simulink model "Mission_Manager_HIL"  (R2025b)
settings: Solver=FixedStepDiscrete  StartTime=0.0  StopTime=tspan  FixedStep=dt_sim  RelTol=1e-3
undefined symbols (not defined in the file): dt_control, dt_data, pwm_zero_set
libraries: ros2lib x7
settings Model: Creator=vulcangrip  LastModifiedBy=kjhaydon
settings OptimizationCC: DefaultParameterBehavior=Inlined  EnhancedBackFolding=on  PassReuseOutputArgsAs=Individual arguments  ZeroExternalMemoryAtStartup=off  ZeroInternalMemoryAtStartup=off  MaxStackSize=64  OptimizeBlockOrder=speed  DifferentSizesBufferReuse=on  OptimizationCustomize=off  EfficientTunableParamExpr=on
settings DebuggingCC: ParameterTunabilityLossMsg=error
settings HardwareCC: ProdBitPerLong=64.0  ProdHWDeviceType=Intel->x86-64 (Linux 64)
settings SFSimCC: MATLABDynamicMemAlloc=off  SimTargetLang=C++  SimDLTargetLibrary=mkl-dnn
settings RTWCC: SystemTargetFile=ert.tlc  HardwareBoard=Robot Operating System 2 (ROS 2)  TLCOptions="-aInlineSetEventsForThisBaseRateFcn=TLC_FALSE -aSuppressMultiTaskScheduler=TLC_FALSE  -aRateBasedStepFcn=0"  GenCodeOnly=on  TemplateMakefile=ert_default_tmf  Toolchain=Colcon Tools  TargetLang=C++  CheckMdlBeforeBuild=Warning  Description=Embedded Coder
settings CodeAppCC: ForceParamTrailComments=on  IgnoreCustomStorageClasses=off  OperatorAnnotations=on  SimulinkDataObjDesc=on  SFDataObjDesc=on  InsertBlockDesc=on
settings ERTTargetCC: ExtModeTransport=2.0  ExtModeStaticAlloc=on  ExtModeAutomaticAllocSize=off  ExtModeMexFile=ext_xcp  ExtModeIntrfLevel=Level2 - Open  RootIOFormat=Structure reference  TargetLangStandard=C++11 (ISO)  CodeInterfacePackaging=C++ class  SubcomponentCodeInterfacePackaging=C++ class

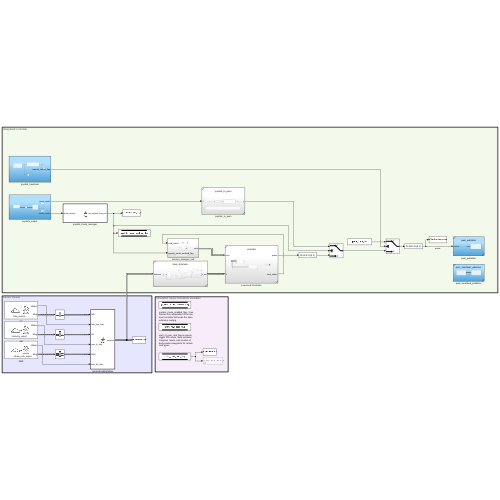
[thumbnail: Simulink's stored preview of the top-level diagram]
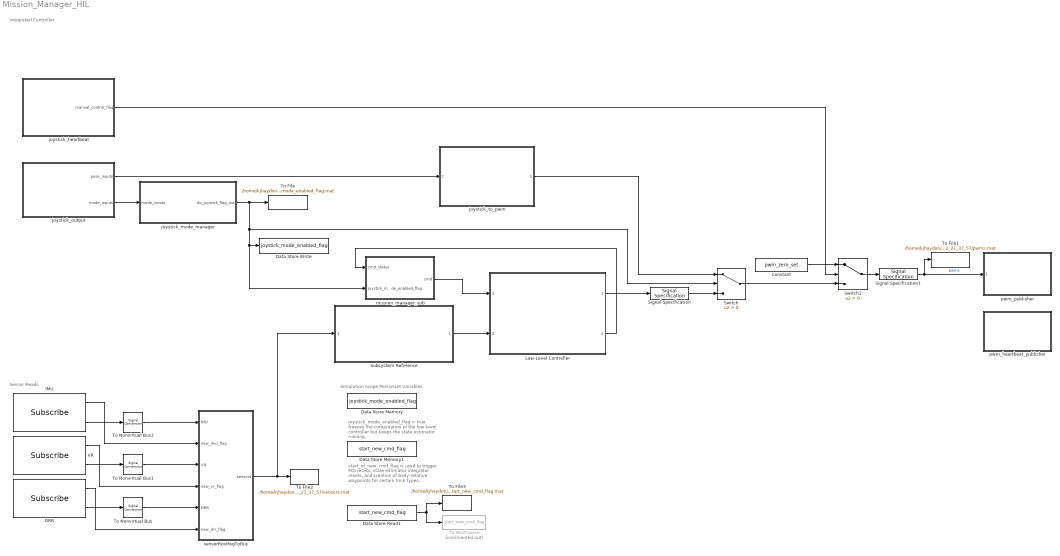
== system Mission_Manager_HIL ==
  note: Integrated Controller
  note: Sensor Reads
  note: Simulation Scope Persistant Variables
  note: joystick_mode_enabled_flag = true freezes the computation of the low-level controller but keeps the state estimator running.
  note: start_of_new_cmd_flag is used to trigger PID resets, state estimator integrator resets, and creation of body-relative waypoints for certain trick types.
  Constant : Constant  Value=pwm_zero_set  OutDataTypeStr=int32
  DRR : ros2lib/Subscribe  topicSource=Select from ROS network  topic=/dead_reck_report  messageType=custom_interfaces/DRR  sampleTime=-1  QOSHistory=Keep last  QOSDepth=10  QOSReliability=Reliable  QOSDurability=Volatile  QOSDeadline=Inf  QOSLifespan=Inf  QOSLiveliness=Automatic  QOSLeaseDuration=Inf  QOSAvoidROSNamespaceConventions=off
  Data Store Memory : DataStoreMemory  DataStoreName=joystick_mode_enabled_flag  WriteAfterWriteMsg=warning  InitialValue=initial_joystick_mode_enabled_flag  ShowAdditionalParam=off  OutDataTypeStr=boolean
  Data Store Memory1 : DataStoreMemory  DataStoreName=start_new_cmd_flag  WriteAfterWriteMsg=warning  InitialValue=true  ShowAdditionalParam=off  OutDataTypeStr=boolean
  Data Store Read1 : DataStoreRead  DataStoreName=start_new_cmd_flag  IndexOptions=Index vector (dialog)  Indices=1  OutputSizes=1
  Data Store Write : DataStoreWrite  DataStoreName=joystick_mode_enabled_flag  SampleTime=dt_control  IndexOptions=Index vector (dialog)  Indices=1  OutputSizes=1
  IMU : ros2lib/Subscribe  topicSource=Specify your own  topic=/imu_custom  messageType=custom_interfaces/Imu  sampleTime=1/100  QOSHistory=Keep last  QOSDepth=10  QOSReliability=Reliable  QOSDurability=Volatile  QOSDeadline=Inf  QOSLifespan=Inf  QOSLiveliness=Automatic  QOSLeaseDuration=Inf  QOSAvoidROSNamespaceConventions=off
  Low-Level Controller : Subsystem  ReferencedSubsystem=controller
  Signal Specification : SignalSpecification  OutDataTypeStr=int32  Dimensions=[8 1]
  Signal Specification1 : SignalSpecification  OutDataTypeStr=int32  Dimensions=[8 1]
  Subsystem Reference : Subsystem  ReferencedSubsystem=State_Estimator
  Switch : Switch  Criteria=u2 > Threshold  SaturateOnIntegerOverflow=off  InputSameDT=off
  Switch1 : Switch  Criteria=u2 > Threshold  SaturateOnIntegerOverflow=off  InputSameDT=off
  To File : ToFile  Filename=/home/kjhaydon/Github/Robosub/SimulinkPlant/data/2026_06_22_21_37_57/joystick_mode_enabled_flag.mat  MatrixName=joystick_mode_enabled_flag  SaveFormat=Timeseries  SampleTime=dt_control
  To File1 : ToFile  Filename=/home/kjhaydon/Github/Robosub/SimulinkPlant/data/2026_06_22_21_37_57/pwms.mat  MatrixName=pwms  SaveFormat=Timeseries  SampleTime=dt_control
  To File2 : ToFile  Filename=/home/kjhaydon/Github/Robosub/SimulinkPlant/data/2026_06_22_21_37_57/sensors.mat  MatrixName=sensors  SaveFormat=Timeseries
  To File3 : ToFile  Filename=/home/kjhaydon/Github/Robosub/SimulinkPlant/data/2026_06_22_21_37_57/start_new_cmd_flag.mat  MatrixName=start_new_cmd_flag  SaveFormat=Timeseries
  To Nonvirtual Bus : SignalConversion  ConversionOutput=Nonvirtual bus  OutDataTypeStr=Bus: SL_Bus_custom_interfaces_DRR  OverrideOpt=off
  To Nonvirtual Bus1 : SignalConversion  ConversionOutput=Nonvirtual bus  OutDataTypeStr=Bus: SL_Bus_custom_interfaces_VR  OverrideOpt=off
  To Nonvirtual Bus2 : SignalConversion  ConversionOutput=Nonvirtual bus  OutDataTypeStr=Bus: SL_Bus_custom_interfaces_Imu  OverrideOpt=off
  To Workspace : ToWorkspace  Commented=on  VariableName=start_new_cmd_flag  SaveFormat=Timeseries  SampleTime=dt_data
  VR : ros2lib/Subscribe  topicSource=Select from ROS network  topic=/velocity_report  messageType=custom_interfaces/VR  sampleTime=-1  QOSHistory=Keep last  QOSDepth=10  QOSReliability=Reliable  QOSDurability=Volatile  QOSDeadline=Inf  QOSLifespan=Inf  QOSLiveliness=Automatic  QOSLeaseDuration=Inf  QOSAvoidROSNamespaceConventions=off
  joystick_heartbeat : Subsystem
  joystick_mode_manager : MATLAB Function  TreatAsAtomicUnit=on
  joystick_output : Subsystem
  joystick_to_pwm : Subsystem  ReferencedSubsystem=joystick_to_pwm
  mission_manager_sub : Subsystem
  pwm_heartbeat_publisher : Subsystem  ReferencedSubsystem=pwm_heartbeat_publisher
  pwm_publisher : Subsystem  ReferencedSubsystem=pwm_publisher
  sensorRosMsgToBus : MATLAB Function  TreatAsAtomicUnit=on
  wires:
  IMU/2 -> To Nonvirtual Bus2/1
  DRR/2 -> To Nonvirtual Bus/1
  VR/2 -> To Nonvirtual Bus1/1
  joystick_output/2(mode_inputs) -> joystick_mode_manager/1(mode_inputs)
  mission_manager_sub/1(cmd) -> Low-Level Controller/1
  Low-Level Controller/2 -> mission_manager_sub/1(cmd_status)
  Low-Level Controller/1 -> Signal Specification/1
  joystick_to_pwm/1 -> Switch/1
  Signal Specification/1 -> Switch/3
  joystick_output/1(pose_inputs) -> joystick_to_pwm/1
  Subsystem Reference/1 -> Low-Level Controller/2
  To Nonvirtual Bus1/1 -> sensorRosMsgToBus/3(VR)
  To Nonvirtual Bus/1 -> sensorRosMsgToBus/5(DRR)
  sensorRosMsgToBus/1(sensors) -> Subsystem Reference/1, To File2/1
  joystick_mode_manager/1(do_joystick_flag_out) -> mission_manager_sub/2(joystick_mode_enabled_flag), Data Store Write/1, Switch/2, To File/1
  Signal Specification1/1 -> To File1/1, pwm_publisher/1  "pwms"
  To Nonvirtual Bus2/1 -> sensorRosMsgToBus/1(IMU)
  Data Store Read1/1 -> To File3/1, To Workspace/1
  joystick_heartbeat/1(manual_control_flag) -> Switch1/2
  Switch1/1 -> Signal Specification1/1
  Switch/1 -> Switch1/3
  Constant/1 -> Switch1/1
  IMU/1 -> sensorRosMsgToBus/2(new_imu_flag)
  VR/1 -> sensorRosMsgToBus/4(new_vr_flag)
  DRR/1 -> sensorRosMsgToBus/6(new_drr_flag)

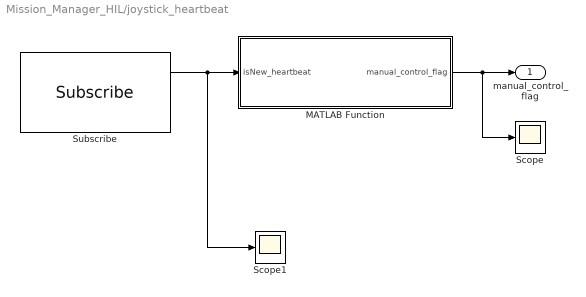
== system Mission_Manager_HIL/joystick_heartbeat ==
  MATLAB Function : MATLAB Function  TreatAsAtomicUnit=on
  Scope : Scope
      settings: ActiveDisplayYMinimum=-0.12499999999999997  ActiveDisplayYMaximum=1.125
  Scope1 : Scope
      settings: ActiveDisplayYMinimum=-0.031272765620221396  ActiveDisplayYMaximum=0.23950064914425354
  Subscribe : ros2lib/Subscribe  topicSource=Select from ROS network  topic=/joystick_heartbeat  messageType=std_msgs/Empty  sampleTime=-1  QOSHistory=Keep last  QOSDepth=10  QOSReliability=Reliable  QOSDurability=Volatile  QOSDeadline=Inf  QOSLifespan=Inf  QOSLiveliness=Automatic  QOSLeaseDuration=Inf  QOSAvoidROSNamespaceConventions=off
  manual_control_flag : Outport
  wires:
  Subscribe/1 -> Scope1/1, MATLAB Function/1(isNew_heartbeat)
  MATLAB Function/1(manual_control_flag) -> Scope/1, manual_control_flag/1

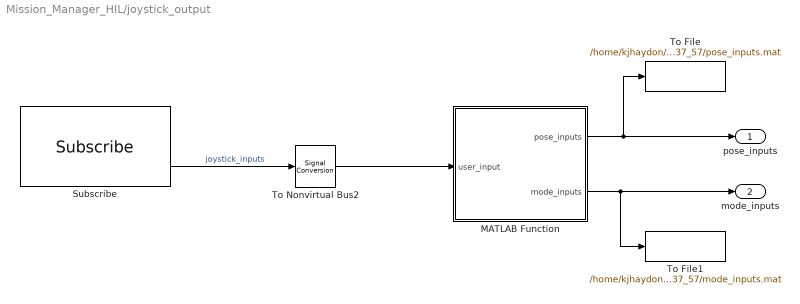
== system Mission_Manager_HIL/joystick_output ==
  MATLAB Function : MATLAB Function  TreatAsAtomicUnit=on
  Subscribe : ros2lib/Subscribe  topicSource=Specify your own  topic=/ps5_controller  messageType=custom_interfaces/Gamepad  sampleTime=1/100  QOSHistory=Keep last  QOSDepth=10  QOSReliability=Reliable  QOSDurability=Volatile  QOSDeadline=Inf  QOSLifespan=Inf  QOSLiveliness=Automatic  QOSLeaseDuration=Inf  QOSAvoidROSNamespaceConventions=off
  To File : ToFile  Filename=/home/kjhaydon/Github/Robosub/SimulinkPlant/data/2026_06_22_21_37_57/pose_inputs.mat  MatrixName=pose_inputs  SaveFormat=Timeseries  SampleTime=dt_control
  To File1 : ToFile  Filename=/home/kjhaydon/Github/Robosub/SimulinkPlant/data/2026_06_22_21_37_57/mode_inputs.mat  MatrixName=mode_inputs  SaveFormat=Timeseries  SampleTime=dt_control
  To Nonvirtual Bus2 : SignalConversion  ConversionOutput=Nonvirtual bus  OutDataTypeStr=Bus: SL_Bus_custom_interfaces_Gamepad  OverrideOpt=off
  pose_inputs : Outport
  mode_inputs : Outport  Port=2
  wires:
  Subscribe/2 -> To Nonvirtual Bus2/1  "joystick_inputs"
  To Nonvirtual Bus2/1 -> MATLAB Function/1(user_input)
  MATLAB Function/1(pose_inputs) -> pose_inputs/1, To File/1
  MATLAB Function/2(mode_inputs) -> To File1/1, mode_inputs/1

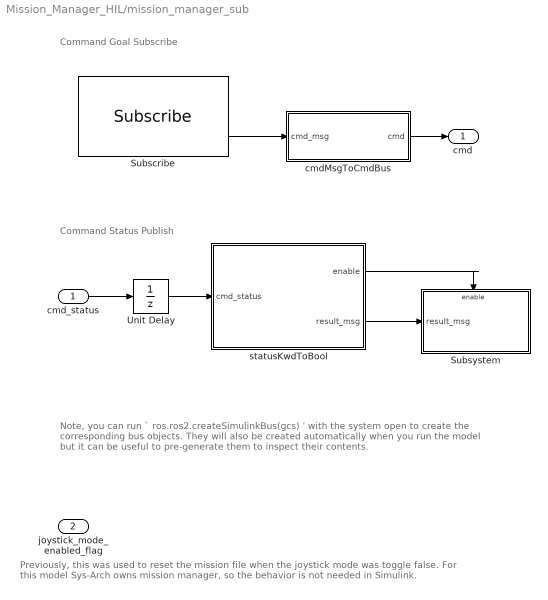
== system Mission_Manager_HIL/mission_manager_sub ==
  note: Note, you can run ` ros.ros2.createSimulinkBus(gcs) ' with the system open to create the
      | corresponding bus objects. They will also be created automatically when you
      | run the model but it can be useful to pre-generate them to inspect their contents.
  note: Command Status Publish
  note: Previously, this was used to reset the mission file when the joystick mode was toggle false. For this model Sys-Arch owns mission manager, so the behavior is not needed in Simulink.
  note: Command Goal Subscribe
  cmd_status : Inport  SampleTime=dt_control
  joystick_mode_enabled_flag : Inport  Port=2
  Subscribe : ros2lib/Subscribe  topicSource=Specify your own  topic=/cmd_message  messageType=custom_interfaces/Goal  sampleTime=dt_control  QOSHistory=Keep last  QOSDepth=10  QOSReliability=Reliable  QOSDurability=Volatile  QOSDeadline=Inf  QOSLifespan=Inf  QOSLiveliness=Automatic  QOSLeaseDuration=Inf  QOSAvoidROSNamespaceConventions=off
  Subsystem : Subsystem
  Unit Delay : UnitDelay  SampleTime=-1  HasFrameUpgradeWarning=on
  cmdMsgToCmdBus : MATLAB Function  TreatAsAtomicUnit=on
  statusKwdToBool : MATLAB Function  TreatAsAtomicUnit=on
  cmd : Outport  SampleTime=dt_control
  wires:
  cmd_status/1 -> Unit Delay/1
  statusKwdToBool/1(enable) -> Subsystem/Enable
  Unit Delay/1 -> statusKwdToBool/1(cmd_status)
  cmdMsgToCmdBus/1(cmd) -> cmd/1
  Subscribe/2 -> cmdMsgToCmdBus/1(cmd_msg)
  statusKwdToBool/2(result_msg) -> Subsystem/1(result_msg)

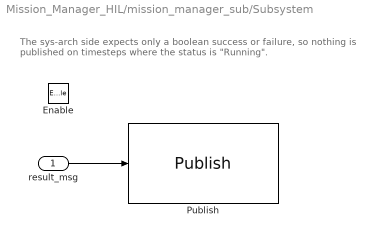
== system Mission_Manager_HIL/mission_manager_sub/Subsystem ==
  note: The sys-arch side expects only a boolean success or failure, so nothing
      | is published on timesteps where the status is "Running".
  result_msg : Inport
  Enable : EnablePort
  Publish : ros2lib/Publish  topicSource=Specify your own  topic=/cmd_result  messageType=custom_interfaces/Result  QOSHistory=Keep last  QOSDepth=10  QOSReliability=Reliable  QOSDurability=Volatile  QOSDeadline=Inf  QOSLifespan=Inf  QOSLiveliness=Automatic  QOSLeaseDuration=Inf  QOSAvoidROSNamespaceConventions=off
  wires:
  result_msg/1 -> Publish/1

== matlab function Mission_Manager_HIL/mission_manager_sub/statusKwdToBool ==
  data: enable output; cmd_status input; result_msg output Bus: SL_Bus_custom_interfaces_Result
function [enable, result_msg]   = fcn(cmd_status)

[enable, result_msg] = statusKwdToBool(cmd_status);

== matlab function Mission_Manager_HIL/joystick_output/MATLAB Function ==
  data: user_input input; pose_inputs output; mode_inputs output
function [pose_inputs, mode_inputs] = fcn(user_input)

[pose_inputs, mode_inputs] = gamepad_parser(user_input);

== matlab function Mission_Manager_HIL/joystick_heartbeat/MATLAB Function ==
  data: isNew_heartbeat input boolean; manual_control_flag output boolean; dt_control parameter
function manual_control_flag = fcn(isNew_heartbeat,dt_control)

manual_control_flag = heartbeat_interpreter(isNew_heartbeat,dt_control);

== matlab function Mission_Manager_HIL/joystick_mode_manager ==
  data: mode_inputs input; do_joystick_flag_out output
function do_joystick_flag_out   = fcn(mode_inputs)
    
[do_joystick_flag_out,~] = mode_manager(mode_inputs);

== matlab function Mission_Manager_HIL/mission_manager_sub/cmdMsgToCmdBus ==
  data: cmd_msg input Bus: SL_Bus_custom_interfaces_Goal; cmd output Bus: cmd_bus
function cmd = fcn(cmd_msg)

cmd = cmdMsgToCmdBus(cmd_msg);

end

== matlab function Mission_Manager_HIL/sensorRosMsgToBus ==
  data: IMU input; new_imu_flag input; sensors output Bus: sensor_bus; VR input; new_vr_flag input; DRR input size=[1,1]; new_drr_flag input
function sensors = fcn(IMU, new_imu_flag, VR, new_vr_flag, DRR, new_drr_flag)

sensors = sensorRosMsgToBus(IMU, new_imu_flag, VR, new_vr_flag, DRR, new_drr_flag);
